simulink model "OBC"  (R2017a)
settings: Solver=VariableStepAuto  StartTime=0.0  StopTime=10.0  RelTol=1e-3
settings Model: Creator=pc  LastModifiedBy=pc

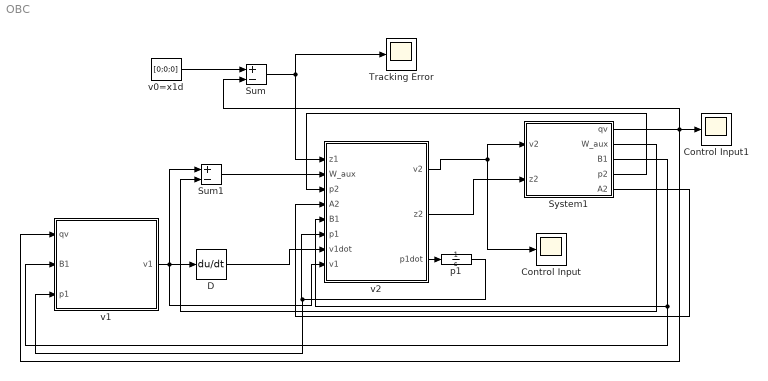
== system OBC ==
  Control Input : Scope
  Control Input1 : Scope
  D : Derivative
  Sum : Sum  Inputs=+-
  Sum1 : Sum  Inputs=+-
  System1 : Subsystem
  Tracking Error : Scope
  p1 : Integrator  InitialCondition=[1 0 0;0 1 0;0 0 1]
  v0=x1d : Constant  Value=[0;0;0]
  v1 : MATLAB Function  TreatAsAtomicUnit=on
  v2 : MATLAB Function  TreatAsAtomicUnit=on
  wires:
  D/1 -> v2/7(v1dot)
  System1/2(W_aux) -> Sum1/2
  System1/1(qv) -> Control Input1/1, v1/1(qv), Sum/2
  v2/1(v2) -> Control Input/1, System1/1(v2)
  Sum1/1 -> v2/2(W_aux)
  v1/1(v1) -> v2/8(v1), Sum1/1, D/1
  v0=x1d/1 -> Sum/1
  Sum/1 -> v2/1(z1), Tracking Error/1
  System1/3(B1) -> v2/5(B1), v1/2(B1)
  v2/3(p1dot) -> p1/1
  p1/1 -> v1/3(p1), v2/6(p1)
  v2/2(z2) -> System1/2(z2)
  System1/4(p2) -> v2/3(p2)
  System1/5(A2) -> v2/4(A2)

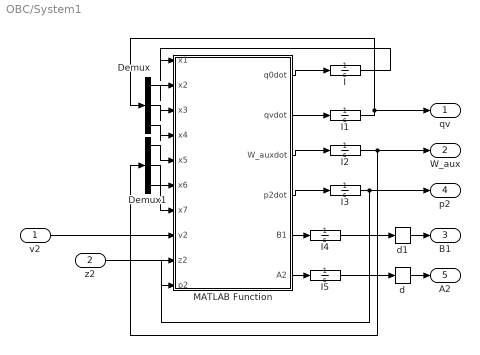
== system OBC/System1 ==
  v2 : Inport
  z2 : Inport  Port=2
  Demux : Demux  Outputs=3
  Demux1 : Demux  Outputs=3
  I : Integrator  InitialCondition=0.8224
  I1 : Integrator  InitialCondition=[0.2226 0.4397 0.3604]'
  I2 : Integrator  InitialCondition=[-1.5 -5.8 -6.8]'
  I3 : Integrator  InitialCondition=[1 0 0;0 1 0;0 0 1]
  I4 : Integrator  InitialCondition=[1 0 0;0 1 0;0 0 1]
  I5 : Integrator  InitialCondition=[1 0 0;0 1 0;0 0 1]
  MATLAB Function : MATLAB Function  TreatAsAtomicUnit=on
  d : Derivative
  d1 : Derivative
  qv : Outport
  W_aux : Outport  Port=2
  B1 : Outport  Port=3
  p2 : Outport  Port=4
  A2 : Outport  Port=5
  wires:
  MATLAB Function/1(q0dot) -> I/1
  I/1 -> MATLAB Function/1(x1)
  v2/1 -> MATLAB Function/8(v2)
  MATLAB Function/2(qvdot) -> I1/1
  MATLAB Function/3(W_auxdot) -> I2/1
  MATLAB Function/4(p2dot) -> I3/1
  I1/1 -> qv/1, Demux/1
  I3/1 -> MATLAB Function/10(p2), p2/1
  Demux/1 -> MATLAB Function/2(x2)
  Demux/2 -> MATLAB Function/3(x3)
  Demux/3 -> MATLAB Function/4(x4)
  Demux1/2 -> MATLAB Function/6(x6)
  Demux1/3 -> MATLAB Function/7(x7)
  Demux1/1 -> MATLAB Function/5(x5)
  I2/1 -> Demux1/1, W_aux/1
  z2/1 -> MATLAB Function/9(z2)
  MATLAB Function/5(B1) -> I4/1
  MATLAB Function/6(A2) -> I5/1
  I4/1 -> d1/1
  I5/1 -> d/1
  d1/1 -> B1/1
  d/1 -> A2/1

== matlab function OBC/v2 ==
  data: z1 input; W_aux input; p2 input; A2 input; B1 input; p1 input; v1dot input; v1 input; v2 output; z2 output; p1dot output
function [v2,z2,p1dot] = fcn(z1,W_aux,p2,A2,B1,p1,v1dot,v1)
Q0=0.8224;
IR2=33.3333*eye(3,3);
R1=0.1*eye(3,3);
Q1=eye(3,3);
gamma= 150;
B2=102.0408*eye(3,3);%equation(20)
v=[0.0098,0.0098,0.0176];
B22=102.0408*eye(3,3);
J=diag(v);
z2=v1-W_aux;
W2=1/(2*gamma^2)*B22'*p2*z2;%equation(88)
p1dot=p1*B1*R1\B1'*p1-Q1;%equation(97)
v2=IR2*B2'*p2*z2+J*v1dot*sign(Q0)-J*A2*v1*sign(Q0)+J*p2\B1'*p1*z1-J*B22*W2;

== matlab function OBC/v1 ==
  data: qv input; v1 output; B1 input; p1 input
function v1 = fcn(qv,B1,p1)
v1=[0;0;0];
Q0=0.8224;
R1=0.1*eye(3,3);
v1=-inv(R1)*B1'*p1*qv*sign(Q0);%equation(84)

== matlab function OBC/System1/MATLAB Function ==
  data: x1 input; x2 input; x3 input; q0dot output; qvdot output; W_auxdot output; x4 input; x5 input; x6 input; x7 input; v2 input; z2 input; p2dot output; p2 input; B1 output; A2 output
function [q0dot,qvdot,W_auxdot,p2dot,B1,A2] = fcn(x1,x2,x3,x4,x5,x6,x7,v2,z2,p2)
Q0=0.8224;
R1=0.1*eye(3,3);
v=[0.0098,0.0098,0.0176];
J=diag(v);
%R2=0.03*eye(3,3);
IR2=33.3333*eye(3,3);
gamma= 150;
Q1=eye(3,3);
Q2=eye(3,3);
B2=102.0408*eye(3,3);%equation(20)
G2=102.0408*eye(3,3);
B22=102.0408*eye(3,3);
W_d=[0;0;0];
%--------------------------------------------------------------------------------------------------------------------
R_T=[ x1^2+x2^2-x3^2-x4^2, 2*(x2*x3+x1*x4), 2*(x2*x4-x1*x3)   
          2*(x2*x3-x1*x4), x1^2-x2^2+x3^2-x4^2, 2*(x3*x4+x1*x2)   
          2*(x2*x4+x1*x3), 2*(x3*x4-x1*x2), x1^2-x2^2-x3^2+x4^2];%equation(9)
W_star=R_T*W_d;
q0=x1;
qv=[x2;x3;x4];
W_aux=[x5;x6;x7];
%--------------------------------------------------------------------------------------------------------------------
B1=0.5*[0,-x4,x3;x4,0,-x2;-x3,x2,0]+q0*eye(3,3);%equation(26.2)
A2=(-B2*[0,-x7,x6;x7,0,-x5;-x6,x5,0]*J-B2*[0,-W_star(3),W_star(2);W_star(3),0,-W_star(1);-W_star(2),W_star(1),0]*J);%equation(20)
W2=1/(2*gamma^2)*B22'*p2*z2;
q0dot=-0.5*qv'*W_aux;%equation(21)
qvdot=B1*W_aux;
W_auxdot=A2*W_aux+B2*v2+B22*W2;%equation(26.2)
T2=1/(2*gamma^2)*G2*(G2')-B2*IR2*B2';%equation(98)
p2dot=-A2'*p2-p2*A2-p2*T2*p2-Q2;%equation(98)
